simulink model "biplex_core_test"  (Simulink 7.4)
settings: Solver=VariableStepDiscrete  StartTime=0.0  StopTime=35000  RelTol=1e-3
libraries: xbsIndex_r4 x1215, casper_library_misc x82, casper_library_delays x14, casper_library_ffts_twiddle x1
(part 23 of 27)

== system biplex_core_test/biplex_core/fft_stage_11/butterfly_direct/twiddle_general_4mult/coeff_gen ==
  rst : Inport
  Counter : xbsIndex_r4/Counter  cnt_type=Free Running  cnt_to=Inf  operation=Up  start_count=0  cnt_by_val=1  arith_type=Unsigned  n_bits=13  bin_pt=0  load_pin=off  rst=on  en=off  explicit_period=on  period=1  dbl_ovrd=off  use_behavioral_HDL=off  implementation=Fabric  block_type=counter
      settings: block_version=11.4
  ROM : xbsIndex_r4/ROM  depth=1024  initVector="[1                                      0                       0.70709228515625                      -0.70709228515625                       0.92388916015625                       -0.3826904296875                        0.3826904296875                      -0.92388916015625                       0.98077392578125                        -0.195068359375                        0.5555419921875                      -0.83148193359375                       0.83148193359375                       -0.5555419921875                         0.195068359375                      -0.98077392578125                       0.99517822265625                       -0.0980224609375                        0.6343994140625                      -0.77301025390625                       0.88189697265625                      -0.47137451171875                         0.290283203125                      -0.95697021484375                       0.95697021484375                        -0.290283203125                       0.47137451171875                      -0.88189697265625                       0.77301025390625                       -0.6343994140625                        0.0980224609375                      -0.99517822265625                         0.998779296875                        -0.049072265625                       0.67156982421875                        -0.740966796875                       0.90399169921875                      -0.42755126953125                           0.3369140625                       -0.9415283203125                       0.97003173828125                      -0.24298095703125                       0.51409912109375                      -0.85772705078125                          0.80322265625                           -0.595703125                         0.146728515625                      -0.98919677734375                       0.98919677734375                        -0.146728515625                            0.595703125                         -0.80322265625                       0.85772705078125                      -0.51409912109375                       0.24298095703125                      -0.97003173828125                        0.9415283203125                          -0.3369140625                       0.42755126953125                      -0.90399169921875                         0.740966796875                      -0.67156982421875                         0.049072265625                        -0.998779296875                       0.99969482421875                       -0.0245361328125                       0.68951416015625                       -0.7242431640625                        0.9141845703125                      -0.40521240234375                       0.35992431640625                       -0.9329833984375                        0.9757080078125                       -0.2191162109375                       0.53497314453125                       -0.8448486328125                       0.81756591796875                       -0.5758056640625                       0.17095947265625                      -0.98529052734375                       0.99249267578125                       -0.1224365234375                            0.615234375                        -0.788330078125                           0.8701171875                        -0.492919921875                        0.2667236328125                      -0.96380615234375                       0.94952392578125                      -0.31365966796875                        0.4495849609375                      -0.89324951171875                        0.7572021484375                       -0.6531982421875                       0.07354736328125                        -0.997314453125                         0.997314453125                      -0.07354736328125                        0.6531982421875                       -0.7572021484375                       0.89324951171875                       -0.4495849609375                       0.31365966796875 ...(+35900 chars)]"  distributed_mem=Block RAM  rst=off  init_reg=0  en=off  latency=2  arith_type="Signed  (2's comp)"  n_bits=16  bin_pt=14  dbl_ovrd=off  optimize=Area  use_rpm=on  block_type=sprom
      settings: block_version=11.4
  ROM1 : xbsIndex_r4/ROM  depth=1024  initVector="[0                                     -1                      -0.70709228515625                      -0.70709228515625                       -0.3826904296875                      -0.92388916015625                      -0.92388916015625                       -0.3826904296875                        -0.195068359375                      -0.98077392578125                      -0.83148193359375                       -0.5555419921875                       -0.5555419921875                      -0.83148193359375                      -0.98077392578125                        -0.195068359375                       -0.0980224609375                      -0.99517822265625                      -0.77301025390625                       -0.6343994140625                      -0.47137451171875                      -0.88189697265625                      -0.95697021484375                        -0.290283203125                        -0.290283203125                      -0.95697021484375                      -0.88189697265625                      -0.47137451171875                       -0.6343994140625                      -0.77301025390625                      -0.99517822265625                       -0.0980224609375                        -0.049072265625                        -0.998779296875                        -0.740966796875                      -0.67156982421875                      -0.42755126953125                      -0.90399169921875                       -0.9415283203125                          -0.3369140625                      -0.24298095703125                      -0.97003173828125                      -0.85772705078125                      -0.51409912109375                           -0.595703125                         -0.80322265625                      -0.98919677734375                        -0.146728515625                        -0.146728515625                      -0.98919677734375                         -0.80322265625                           -0.595703125                      -0.51409912109375                      -0.85772705078125                      -0.97003173828125                      -0.24298095703125                          -0.3369140625                       -0.9415283203125                      -0.90399169921875                      -0.42755126953125                      -0.67156982421875                        -0.740966796875                        -0.998779296875                        -0.049072265625                       -0.0245361328125                      -0.99969482421875                       -0.7242431640625                      -0.68951416015625                      -0.40521240234375                       -0.9141845703125                       -0.9329833984375                      -0.35992431640625                       -0.2191162109375                       -0.9757080078125                       -0.8448486328125                      -0.53497314453125                       -0.5758056640625                      -0.81756591796875                      -0.98529052734375                      -0.17095947265625                       -0.1224365234375                      -0.99249267578125                        -0.788330078125                           -0.615234375                        -0.492919921875                          -0.8701171875                      -0.96380615234375                       -0.2667236328125                      -0.31365966796875                      -0.94952392578125                      -0.89324951171875                       -0.4495849609375                       -0.6531982421875                       -0.7572021484375                        -0.997314453125                      -0.07354736328125                      -0.07354736328125                        -0.997314453125                       -0.7572021484375                       -0.6531982421875                       -0.4495849609375                      -0.89324951171875                      -0.94952392578125 ...(+35900 chars)]"  distributed_mem=Block RAM  rst=off  init_reg=0  en=off  latency=2  arith_type="Signed  (2's comp)"  n_bits=16  bin_pt=14  dbl_ovrd=off  optimize=Area  use_rpm=on  block_type=sprom
      settings: block_version=11.4
  Slice : xbsIndex_r4/Slice  nbits=10  boolean_output=off  mode=Upper Bit Location + Width  bit1=0  base1=MSB of Input  bit0=0  base0=LSB of Input  dbl_ovrd=off  block_type=slice
  ri_to_c : casper_library_misc/ri_to_c  SystemSampleTime=-1
  w : Outport
  wires:
  ri_to_c/1 -> w/1
  rst/1 -> Counter/1
  Counter/1 -> Slice/1
  Slice/1 -> ROM/1, ROM1/1
  ROM/1 -> ri_to_c/1
  ROM1/1 -> ri_to_c/2
